simulink model "VL6112"  (R2022b)
settings: Solver=VariableStepAuto  StartTime=0.0  StopTime=100  RelTol=1e-3
values from neighbouring files (symbols this model uses):
  densityHydrogen = poutlet*(molarMassHydrogen/1000)/(universalGasConstant2*0.001)/OperatingTemperature    (= 0.0969930238153)    [ValveSetData.m]
  flowCoefficientValve = 1.156 * 0.32    (= 0.36992)    [ValveSetData.m]
  hysteresisValve = 0.15    [ValveSetData.m]
  N2 = 6950    [ValveSetData.m]
  OperatingTemperature = T_S+27    (= 300)    [ValveSetData.m]
  pinlet = 12    [ValveSetData.m]
  poutlet = 1.2    [ValveSetData.m]
  responseTimeValve = 0.03    [ValveSetData.m]
  SpecificGravityHydrogen = 0.0696    [ValveSetData.m]
libraries: simulink x1
settings Model: Creator=debjani.ghosh  LastModifiedBy=debjani.ghosh
settings DataIOCC: ReturnWorkspaceOutputs=off

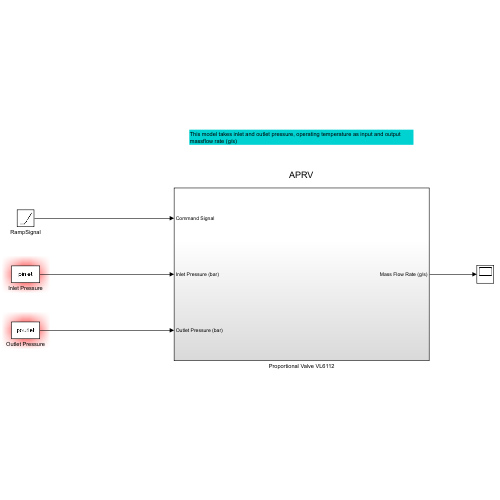
[thumbnail: Simulink's stored preview of the top-level diagram]
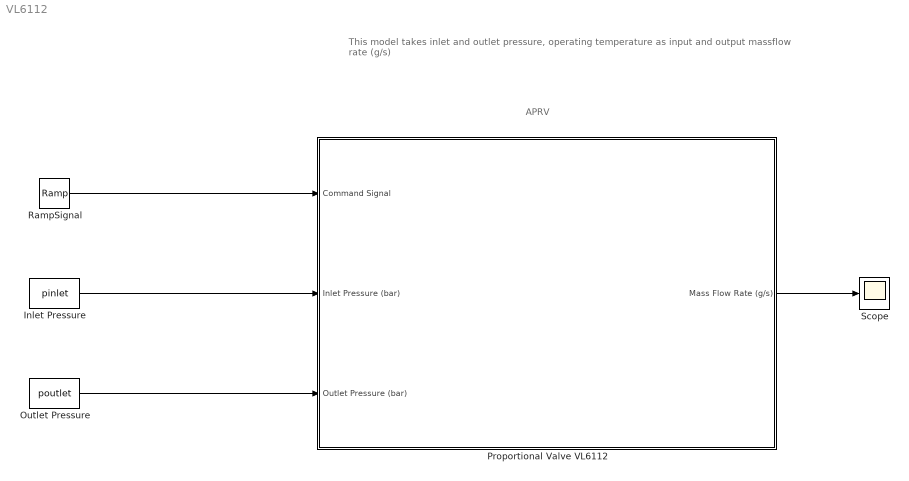
== system VL6112 ==
  note: This model takes inlet and outlet pressure, operating temperature as input and output massflow rate (g/s)
  note: APRV
  Inlet Pressure : Constant  Value=pinlet
  Outlet Pressure : Constant  Value=poutlet
  Proportional Valve VL6112 : Subsystem
  RampSignal : simulink/Sources/Ramp  slope=1/100  start=0  InitialOutput=0
  Scope : Scope
  wires:
  Inlet Pressure/1 -> Proportional Valve VL6112/2(Inlet Pressure (bar))
  Outlet Pressure/1 -> Proportional Valve VL6112/3(Outlet Pressure (bar))
  RampSignal/1 -> Proportional Valve VL6112/1("Command Signal ")
  Proportional Valve VL6112/1(Mass Flow Rate (g/s)) -> Scope/1

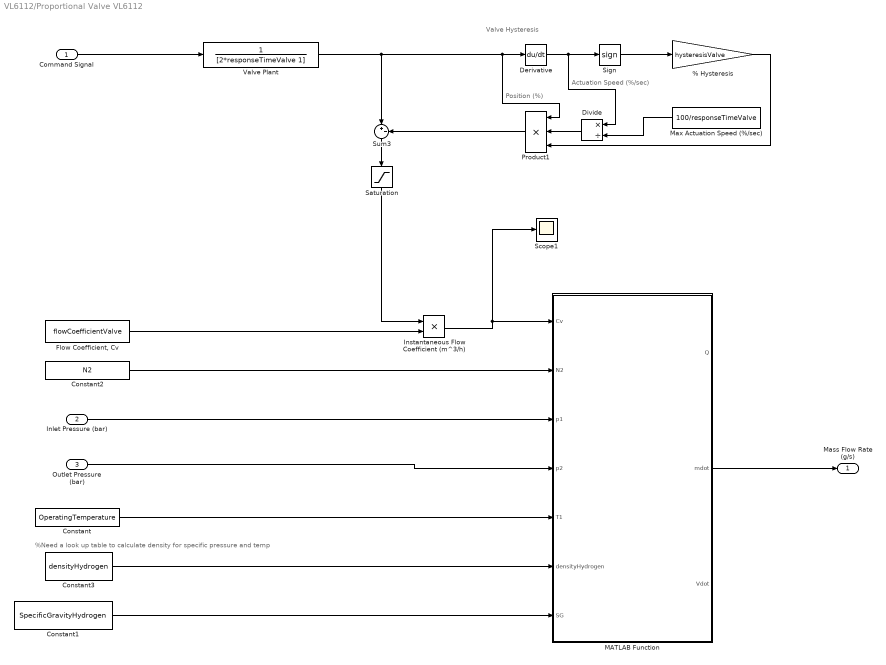
== system VL6112/Proportional Valve VL6112 ==
  note: %Need a look up table to calculate density for specific pressure and temp
  note: Actuation Speed (%/sec)
  note: Position (%)
  note: Valve Hysteresis
  "Command Signal " : Inport
  Inlet Pressure (bar) : Inport  Port=2
  Outlet Pressure (bar) : Inport  Port=3
  % Hysteresis : Gain  Gain=hysteresisValve
  Constant : Constant  Value=OperatingTemperature
  Constant1 : Constant  Value=SpecificGravityHydrogen
  Constant2 : Constant  Value=N2
  Constant3 : Constant  Value=densityHydrogen
  Derivative : Derivative
  Divide : Product  Inputs=*/
  "Flow Coefficient, Cv" : Constant  Value=flowCoefficientValve
  Instantaneous Flow Coefficient (m^3/h) : Product
  MATLAB Function : MATLAB Function  TreatAsAtomicUnit=on
  Max Actuation Speed (%/sec) : Constant  Value=100/responseTimeValve
  Product1 : Product  Inputs=3
  Saturation : Saturate  UpperLimit=1  LowerLimit=0  LinearizeAsGain=off
  Scope1 : Scope
  Sign : Signum  ZeroCross=off
  Sum3 : Sum  Inputs=|+-
  Valve Plant : TransferFcn  Denominator=[2*responseTimeValve 1]
  Mass Flow Rate (g/s) : Outport
  wires:
  Sign/1 -> % Hysteresis/1
  Derivative/1 -> Divide/1, Sign/1
  "Flow Coefficient, Cv"/1 -> Instantaneous Flow Coefficient (m^3/h)/2
  % Hysteresis/1 -> Product1/3
  Product1/1 -> Sum3/2
  Sum3/1 -> Saturation/1
  Divide/1 -> Product1/2
  Max Actuation Speed (%/sec)/1 -> Divide/2
  Instantaneous Flow Coefficient (m^3/h)/1 -> Scope1/1, MATLAB Function/1(Cv)
  Valve Plant/1 -> Sum3/1, Derivative/1, Product1/1
  "Command Signal "/1 -> Valve Plant/1
  MATLAB Function/2(mdot) -> Mass Flow Rate (g/s)/1
  Saturation/1 -> Instantaneous Flow Coefficient (m^3/h)/1
  Constant1/1 -> MATLAB Function/7(SG)
  Constant/1 -> MATLAB Function/5(T1)
  Outlet Pressure (bar)/1 -> MATLAB Function/4(p2)
  Inlet Pressure (bar)/1 -> MATLAB Function/3(p1)
  Constant2/1 -> MATLAB Function/2(N2)
  Constant3/1 -> MATLAB Function/6(densityHydrogen)

== matlab function VL6112/Proportional Valve VL6112/MATLAB Function ==
  data: Q output; Cv input; N2 input; p1 input; p2 input; T1 input; densityHydrogen input; mdot output; SG input; Vdot output
function [Q,mdot, Vdot]   = fcn(Cv, N2, p1,p2, T1,densityHydrogen, SG)
%Calculation of mass flow based on Swagelok 
% Valve Sizing Technical Bulletin


%Calculate pressure difference between inlet and outlet

dp = p1-p2;

if p2 > p1/2

     % low pressure drop - subsonic flow

    Q = N2*Cv*p1*(1-(2*dp)/(3*p1))*sqrt(dp/(p1*SG*T1)); % standard volumetric flow rate in lpm 

else
   
    % high pressure drop - sonic flow (independent of downstream pressure)

    Q =  0.471*N2*Cv*p1*sqrt(1/(SG*T1)); % standard volumetric flow rate in lpm  

end

   %Comment: densityHydrogen must be a value dependent on operating T and p

    mdot = 0.06* Q * densityHydrogen* 1000/3600;  %g/s

    %Volumetric flow rate in lpm @ operating T and p
    % T1=T2

    Vdot = Q * 1.01 * T1 /( p2 * 273);  % lpm
